simulink model "Motor_Param_Est"  (R2017a)
settings: Solver=ode15s  StartTime=0.0  StopTime=4  RelTol=1e-3  EnableMultiTasking=on
PreLoadFcn:
  | load Motor_Param_Est_Data;
PostLoadFcn:
  | sn_motor_params_setparams('Initial');
undefined symbols (not defined in the file or in its folder): DC_Motor_J
libraries: fl_lib x6, nesl_utility x3, elec_lib x2
CloseFcn:
  | clear simlog_Motor_Param_Est
Description:
  | Copyright 2014-2018 The MathWorks, Inc.
settings Model: Creator=smiller  LastModifiedBy=smiller
settings DataIOCC: ExternalInput=[Motor_Input_time, Motor_Input_Signal]  LimitDataPoints=on  MaxDataPoints=10000  LoadExternalInput=on  SaveFormat=Array  SignalLoggingName=logsout_Motor_Param_Est
settings OptimizationCC: ExpressionDepthLimit=2147483647  InitFltsAndDblsToZero=on  LifeSpan=inf
settings DebuggingCC: UnderspecifiedInitializationDetection=Classic  MergeDetectMultiDrivingBlocksExec=none  FcnCallInpInsideContextMsg=warning  AllowSymbolicDim=off  StateNameClashWarn=warning  SFUnexpectedBacktrackingDiag=warning  SFNoUnconditionalDefaultTransitionDiag=warning  SFExecutionAtInitializationDiag=none
settings HardwareCC: ProdBitPerPointer=32  ProdBitPerSizeT=32  ProdBitPerPtrDiffT=32  ProdLargestAtomicFloat=None  ProdIntDivRoundTo=Undefined  ProdEndianess=Unspecified  ProdWordSize=32  ProdHWDeviceType=32-bit Generic
settings ModelReferenceCC: PropagateSignalLabelsOutOfModel=off
settings GRTTargetCC: TargetLangStandard=C89/C90 (ANSI)  GeneratePreprocessorConditionals=Disable all  CombineOutputUpdateFcns=off  GRTInterface=on
settings ConfigComp: CovMetricSettings=dw  CovHtmlReporting=on  CovSaveCumulativeToWorkspaceVar=on  CovSaveSingleToWorkspaceVar=on  CovExternalEMLEnable=off  CovSFcnEnable=off
settings SimscapeCC: SimscapeLogType=all  SimscapeLogSimulationStatistics=on  SimscapeLogName=simlog_Motor_Param_Est  SimscapeLogDataHistory=10000

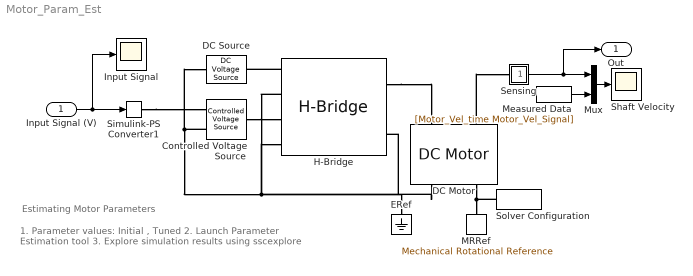
== system Motor_Param_Est ==
  note: 1. Parameter values: Initial , Tuned
      | 2. Launch Parameter Estimation tool
      | 3. Explore simulation results using sscexplore
  note: Estimating Motor Parameters
  Input Signal (V) : Inport
  Controlled Voltage Source : fl_lib/Electrical/Electrical Sources/Controlled Voltage Source
  DC Motor : elec_lib/Actuators & Drivers/Rotational Actuators/DC Motor  parameterization=1  Ra=DC_Motor_R Ohm  La=DC_Motor_L H  emf_or_torque=1  Kv=DC_Motor_K V/(rad/s)  Ki=6.876e-04 N*m/A  T_stall=2.4e-04 N*m  w_max=4000 rpm  w_rated=2500 rpm  P_rated=10 W  V_rated=12 V  J=DC_Motor_J kg*m^2  lam_param=1  lam=DC_Motor_B N*m/(rad/s)  i_noload=0 A  V_i_noload=1.5 V  speed0=0 rpm  alpha=0.00393 1/K  Tmeas=25 degC  thermal_mass=100 J/K  initial_temperature=25 degC
  DC Source : fl_lib/Electrical/Electrical Sources/DC Voltage Source  v0=2.5 V
  ERef : fl_lib/Electrical/Electrical Elements/Electrical Reference
  H-Bridge : elec_lib/Actuators & Drivers/Drivers/H-Bridge  Venable=2.5 V  Vmax=5 V  Vreverse=2.5 V  Vbrake=2.5 V  Vm=12 V  pwm_or_av=2  discontinuous=0  freewheeling_mode=1  freewheeling_mode_disc=1  Ron=0.1 Ohm  Don=0.1 Ohm  Rload=10 Ohm  Lload=1e-5 H  F=10 kHz  thermal_mass=100 J/K  initial_temperature=298.15 K  Ron2=0.1 Ohm  Don2=0.05 Ohm  Tmeas=298.15 K  Tmeas2=398.15 K
      settings: SourceProductName=Simscape Electronics  SourceProductBaseCode=SN
  Input Signal : Scope
  MRRef : fl_lib/Mechanical/Rotational Elements/Mechanical Rotational Reference
  Measured Data : FromWorkspace  VariableName=[Motor_Vel_time Motor_Vel_Signal]  SampleTime=0
  Mux : Mux  Inputs=2
  Sensing : Subsystem
      mask Display: disp('S');
  Shaft Velocity : Scope
  Simulink-PS Converter1 : nesl_utility/Simulink-PS Converter  PhysicalDomain=network_engine_domain  SubClassName=ps_input  LeftPortType=input  RightPortType=output  PseudoPeriodic=off  Frequencies=[]  NoiseDistribution=none  NoiseParameters=[]  Unit=1  AffineConversion=off  FilteringAndDerivatives=zero  SimscapeFilterOrder=1  InputFilterTimeConstant=.001  UdotUserProvided=0
  Solver Configuration : nesl_utility/Solver Configuration  PhysicalDomain=network_engine_domain  SubClassName=solver  LeftPortType=input  RightPortType=generic  Accelerate=off  Tones=[]  Harmonics=[]  SimulateNoise=off  Profile=off  UseLocalSampling=off  EnableSwitchedLinearOptims=on  FrequencyDomain=off  UseCCode=off  RelTol=0.001  AbsTol=1e-06  MinStep=1e-09  ToWorkspace=off  RevertToSquareIcSolve=off  NumHomotopyIterations=100  PhasorMode=off  PhasorModeNumHarmonics=1  OverrideAbsTol=off  DoDC=off  ResidualTolerance=1e-9  UseLocalSolver=off  LocalSolverChoice=NE_BACKWARD_EULER_ADVANCER  LocalSolverSampleTime=.001  DoFixedCost=off  MaxNonlinIter=12  MaxModeIter=2  LinearAlgebra=Sparse  DelaysMemoryBudget=1024  AutomaticFiltering=on  FilteringTimeConstant=0.001
  Out : Outport
  wires:
  Input Signal (V)/1 -> Simulink-PS Converter1/1, Input Signal/1
  Mux/1 -> Shaft Velocity/1
  Measured Data/1 -> Mux/2
  Sensing/1(RPM) -> Mux/1, Out/1
  connections:
  DC Motor/RConn2 -- Solver Configuration/RConn1 -- MRRef/LConn1
  H-Bridge/LConn1 -- DC Source/LConn1
  Simulink-PS Converter1/RConn1 -- Controlled Voltage Source/RConn1
  Controlled Voltage Source/LConn1 -- H-Bridge/LConn3
  H-Bridge/RConn1 -- DC Motor/LConn1
  Controlled Voltage Source/RConn2 -- DC Source/RConn1 -- ERef/LConn1 -- H-Bridge/RConn2 -- DC Motor/RConn1 -- H-Bridge/LConn4 -- H-Bridge/LConn2
  DC Motor/LConn2 -- Sensing/LConn1

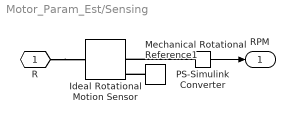
== system Motor_Param_Est/Sensing ==
  Ideal Rotational Motion Sensor : fl_lib/Mechanical/Mechanical Sensors/Ideal Rotational Motion Sensor  offset=0 deg
  Mechanical Rotational Reference1 : fl_lib/Mechanical/Rotational Elements/Mechanical Rotational Reference
  PS-Simulink Converter : nesl_utility/PS-Simulink Converter  PhysicalDomain=network_engine_domain  SubClassName=ps_output  LeftPortType=input  RightPortType=output  PseudoPeriodic=off  Frequencies=[]  Unit=1  AffineConversion=off
  R : PMIOPort  Port=1  Side=Left
  RPM : Outport
  wires:
  PS-Simulink Converter/1 -> RPM/1
  connections:
  PS-Simulink Converter/LConn1 -- Ideal Rotational Motion Sensor/RConn2
  R/RConn1 -- Ideal Rotational Motion Sensor/LConn1
  Mechanical Rotational Reference1/LConn1 -- Ideal Rotational Motion Sensor/RConn1
